simulink model "modelo_robot_6dof_dininv"  (R2023b)
settings: Solver=ode45  StartTime=0.0  StopTime=tsim  FixedStep=tstep  MaxStep=tstep
undefined symbols (not defined in the file): robot_params, tr_ref
(part 1 of 2)
settings Model: Creator=HP  LastModifiedBy=HP

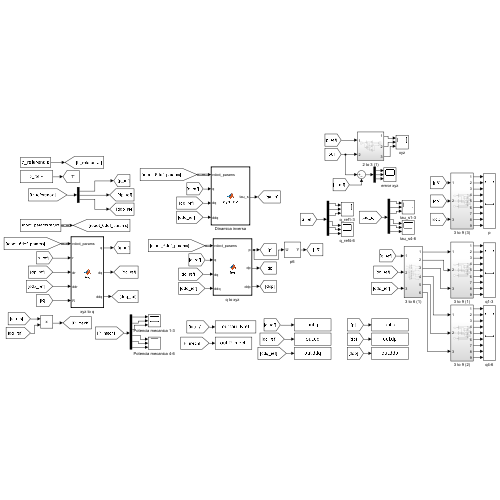
[thumbnail: Simulink's stored preview of the top-level diagram]
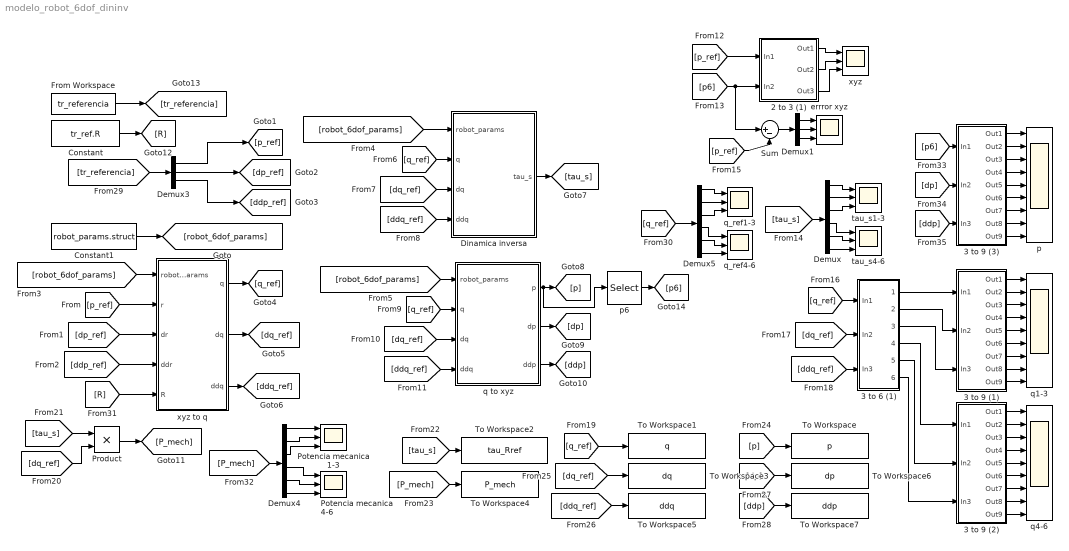
== system modelo_robot_6dof_dininv ==
  2 to 3 (1) : Subsystem
  3 to 6 (1) : Subsystem
  3 to 9 (1) : Subsystem
  3 to 9 (2) : Subsystem
  3 to 9 (3) : Subsystem
  Constant : Constant  Value=tr_ref.R
  Constant1 : Constant  Value=robot_params.struct  OutDataTypeStr=Bus: robot_params_bus
  Demux : Demux  Outputs=6
  Demux1 : Demux  Outputs=3
  Demux3 : Demux  Outputs=3
  Demux4 : Demux  Outputs=6
  Demux5 : Demux  Outputs=6
  Dinamica inversa : MATLAB Function  TreatAsAtomicUnit=on
  From Workspace : FromWorkspace  VariableName=tr_referencia
  Potencia mecanica 1-3 : Scope  NumInputPorts=3
  Potencia mecanica 4-6 : Scope  NumInputPorts=3
  Product : Product
  Sum : Sum  Inputs=|+-
  To Workspace : ToWorkspace  VariableName=p  SaveFormat=Timeseries  SampleTime=-1
  To Workspace1 : ToWorkspace  VariableName=q  SaveFormat=Timeseries  SampleTime=-1
  To Workspace2 : ToWorkspace  VariableName=tau_Rref  SaveFormat=Timeseries  SampleTime=-1
  To Workspace3 : ToWorkspace  VariableName=dq  SaveFormat=Timeseries  SampleTime=-1
  To Workspace4 : ToWorkspace  VariableName=P_mech  SaveFormat=Timeseries  SampleTime=-1
  To Workspace5 : ToWorkspace  VariableName=ddq  SaveFormat=Timeseries  SampleTime=-1
  To Workspace6 : ToWorkspace  VariableName=dp  SaveFormat=Timeseries  SampleTime=-1
  To Workspace7 : ToWorkspace  VariableName=ddp  SaveFormat=Timeseries  SampleTime=-1
  errror xyz : Scope  NumInputPorts=3
  p : Scope  NumInputPorts=9
  p6 : Selector  NumberOfDimensions=2  InputPortWidth=3  IndexOptions=Index vector (dialog),Index vector (dialog)  Indices=[1:3],3  OutputSizes=1,1
  q to xyz : MATLAB Function  TreatAsAtomicUnit=on
  q1-3 : Scope  NumInputPorts=9
  q4-6 : Scope  NumInputPorts=9
  q_ref1-3 : Scope  NumInputPorts=3
  q_ref4-6 : Scope  NumInputPorts=3
  tau_s1-3 : Scope  NumInputPorts=3
  tau_s4-6 : Scope  NumInputPorts=3
  xyz : Scope  NumInputPorts=3
  xyz to q : MATLAB Function  TreatAsAtomicUnit=on
  wires:
  Constant1/1 -> [robot_6dof_params]
  [robot_6dof_params] -> xyz to q/1(robot_params)
  [robot_6dof_params] -> Dinamica inversa/1(robot_params)
  [robot_6dof_params] -> q to xyz/1(robot_params)
  [p_ref] -> xyz to q/2(r)
  [dp_ref] -> xyz to q/3(dr)
  [ddp_ref] -> xyz to q/4(ddr)
  xyz to q/1(q) -> [q_ref]
  xyz to q/2(dq) -> [dq_ref]
  xyz to q/3(ddq) -> [ddq_ref]
  [q_ref] -> Dinamica inversa/2(q)
  [dq_ref] -> Dinamica inversa/3(dq)
  [ddq_ref] -> Dinamica inversa/4(ddq)
  [q_ref] -> q to xyz/2(q)
  [dq_ref] -> q to xyz/3(dq)
  [ddq_ref] -> q to xyz/4(ddq)
  Dinamica inversa/1(tau_s) -> [tau_s]
  q to xyz/3(ddp) -> [ddp]
  q to xyz/2(dp) -> [dp]
  [p_ref] -> 2 to 3 (1)/1(In1)
  2 to 3 (1)/1(Out1) -> xyz/1
  2 to 3 (1)/2(Out2) -> xyz/2
  2 to 3 (1)/3(Out3) -> xyz/3
  [tau_s] -> Demux/1
  Demux/1 -> tau_s1-3/1
  Demux/2 -> tau_s1-3/2
  Demux/3 -> tau_s1-3/3
  [p_ref] -> Sum/2
  Sum/1 -> Demux1/1
  Demux1/1 -> errror xyz/1
  Demux1/2 -> errror xyz/2
  Demux1/3 -> errror xyz/3
  [p6] -> Sum/1, 2 to 3 (1)/2(In2)
  3 to 9 (1)/1(Out1) -> q1-3/1
  3 to 9 (1)/2(Out2) -> q1-3/2
  3 to 9 (1)/3(Out3) -> q1-3/3
  3 to 9 (1)/4(Out4) -> q1-3/4
  3 to 9 (1)/5(Out5) -> q1-3/5
  3 to 9 (1)/6(Out6) -> q1-3/6
  3 to 9 (1)/7(Out7) -> q1-3/7
  3 to 9 (1)/8(Out8) -> q1-3/8
  3 to 9 (1)/9(Out9) -> q1-3/9
  [tau_s] -> Product/1
  [dq_ref] -> Product/2
  [q_ref] -> To Workspace1/1
  [tau_s] -> To Workspace2/1
  Product/1 -> [P_mech]
  [P_mech] -> To Workspace4/1
  [p] -> To Workspace/1
  [dq_ref] -> To Workspace3/1
  [ddq_ref] -> To Workspace5/1
  [dp] -> To Workspace6/1
  [ddp] -> To Workspace7/1
  [tr_referencia] -> Demux3/1
  From Workspace/1 -> [tr_referencia]
  Demux3/1 -> [p_ref]
  Demux3/2 -> [dp_ref]
  Demux3/3 -> [ddp_ref]
  Constant/1 -> [R]
  [R] -> xyz to q/5(R)
  Demux/4 -> tau_s4-6/1
  Demux/5 -> tau_s4-6/2
  Demux/6 -> tau_s4-6/3
  Demux5/1 -> q_ref1-3/1
  Demux5/3 -> q_ref1-3/3
  Demux5/4 -> q_ref4-6/1
  Demux5/5 -> q_ref4-6/2
  Demux5/2 -> q_ref1-3/2
  Demux5/6 -> q_ref4-6/3
  [q_ref] -> Demux5/1
  3 to 9 (2)/1(Out1) -> q4-6/1
  3 to 9 (2)/9(Out9) -> q4-6/9
  3 to 9 (2)/4(Out4) -> q4-6/4
  3 to 9 (2)/6(Out6) -> q4-6/6
  3 to 9 (2)/8(Out8) -> q4-6/8
  3 to 9 (2)/7(Out7) -> q4-6/7
  3 to 9 (2)/3(Out3) -> q4-6/3
  3 to 9 (2)/2(Out2) -> q4-6/2
  3 to 9 (2)/5(Out5) -> q4-6/5
  [q_ref] -> 3 to 6 (1)/1(In1)
  [dq_ref] -> 3 to 6 (1)/2(In2)
  [ddq_ref] -> 3 to 6 (1)/3(In3)
  3 to 6 (1)/1(Out1) -> 3 to 9 (1)/1(In1)
  3 to 6 (1)/2(Out2) -> 3 to 9 (1)/2(In2)
  3 to 6 (1)/3(Out3) -> 3 to 9 (1)/3(In3)
  3 to 6 (1)/4(Out4) -> 3 to 9 (2)/1(In1)
  3 to 6 (1)/5(Out5) -> 3 to 9 (2)/2(In2)
  3 to 6 (1)/6(Out6) -> 3 to 9 (2)/3(In3)
  Demux4/1 -> Potencia mecanica 1-3/1
  Demux4/2 -> Potencia mecanica 1-3/2
  Demux4/3 -> Potencia mecanica 1-3/3
  Demux4/4 -> Potencia mecanica 4-6/1
  Demux4/5 -> Potencia mecanica 4-6/2
  Demux4/6 -> Potencia mecanica 4-6/3
  [P_mech] -> Demux4/1
  p6/1 -> [p6]
  q to xyz/1(p) -> p6/1, [p]
  [p6] -> 3 to 9 (3)/1(In1)
  3 to 9 (3)/7(Out7) -> p/7
  3 to 9 (3)/8(Out8) -> p/8
  3 to 9 (3)/5(Out5) -> p/5
  3 to 9 (3)/1(Out1) -> p/1
  3 to 9 (3)/3(Out3) -> p/3
  3 to 9 (3)/4(Out4) -> p/4
  3 to 9 (3)/9(Out9) -> p/9
  3 to 9 (3)/2(Out2) -> p/2
  [dp] -> 3 to 9 (3)/2(In2)
  [ddp] -> 3 to 9 (3)/3(In3)
  3 to 9 (3)/6(Out6) -> p/6

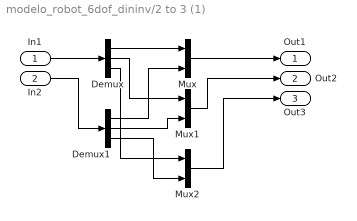
== system modelo_robot_6dof_dininv/2 to 3 (1) ==
  In1 : Inport
  In2 : Inport  Port=2
  Demux : Demux  Outputs=3
  Demux1 : Demux  Outputs=3
  Mux : Mux  Inputs=2
  Mux1 : Mux  Inputs=2
  Mux2 : Mux  Inputs=2
  Out1 : Outport
  Out2 : Outport  Port=2
  Out3 : Outport  Port=3
  wires:
  Demux/3 -> Mux2/1
  Mux2/1 -> Out3/1
  Mux1/1 -> Out2/1
  Demux/1 -> Mux/1
  Demux1/1 -> Mux/2
  In1/1 -> Demux/1
  Demux/2 -> Mux1/1
  Demux1/2 -> Mux1/2
  Mux/1 -> Out1/1
  Demux1/3 -> Mux2/2
  In2/1 -> Demux1/1

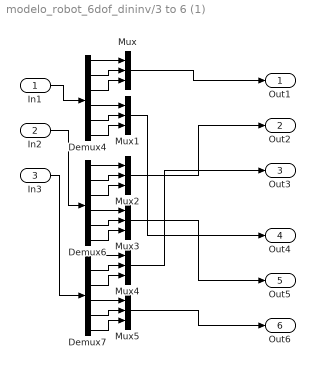
== system modelo_robot_6dof_dininv/3 to 6 (1) ==
  In1 : Inport
  In2 : Inport  Port=2
  In3 : Inport  Port=3
  Demux4 : Demux  Outputs=6
  Demux6 : Demux  Outputs=6
  Demux7 : Demux  Outputs=6
  Mux{,1..5} (6 alike) : Mux  Inputs=3
  Out1 : Outport
  Out2 : Outport  Port=2
  Out3 : Outport  Port=3
  Out4 : Outport  Port=4
  Out5 : Outport  Port=5
  Out6 : Outport  Port=6
  wires:
  Demux6/1 -> Mux2/1
  Demux6/3 -> Mux2/3
  Demux4/2 -> Mux/2
  Demux6/6 -> Mux3/3
  Demux6/2 -> Mux2/2
  Demux6/5 -> Mux3/2
  Mux/1 -> Out1/1
  In1/1 -> Demux4/1
  Demux6/4 -> Mux3/1
  Demux4/1 -> Mux/1
  Demux4/6 -> Mux1/3
  Demux4/4 -> Mux1/1
  Demux7/5 -> Mux5/2
  Demux4/3 -> Mux/3
  Demux4/5 -> Mux1/2
  Demux7/3 -> Mux4/3
  Demux7/1 -> Mux4/1
  Demux7/2 -> Mux4/2
  In3/1 -> Demux7/1
  Mux2/1 -> Out2/1
  Demux7/4 -> Mux5/1
  Demux7/6 -> Mux5/3
  In2/1 -> Demux6/1
  Mux5/1 -> Out6/1
  Mux1/1 -> Out4/1
  Mux4/1 -> Out3/1
  Mux3/1 -> Out5/1

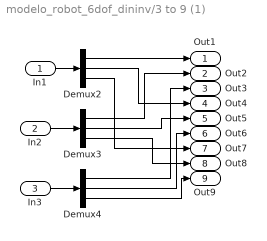
== system modelo_robot_6dof_dininv/3 to 9 (1) ==
  In1 : Inport
  In2 : Inport  Port=2
  In3 : Inport  Port=3
  Demux2 : Demux  Outputs=3
  Demux3 : Demux  Outputs=3
  Demux4 : Demux  Outputs=3
  Out1 : Outport
  Out2 : Outport  Port=2
  Out3 : Outport  Port=3
  Out4 : Outport  Port=4
  Out5 : Outport  Port=5
  Out6 : Outport  Port=6
  Out7 : Outport  Port=7
  Out8 : Outport  Port=8
  Out9 : Outport  Port=9
  wires:
  In3/1 -> Demux4/1
  Demux4/1 -> Out3/1
  Demux2/1 -> Out1/1
  Demux3/3 -> Out8/1
  Demux3/2 -> Out5/1
  Demux3/1 -> Out2/1
  In1/1 -> Demux2/1
  Demux2/3 -> Out7/1
  Demux4/3 -> Out9/1
  Demux4/2 -> Out6/1
  Demux2/2 -> Out4/1
  In2/1 -> Demux3/1

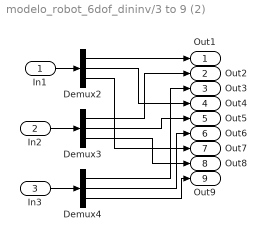
== system modelo_robot_6dof_dininv/3 to 9 (2) ==
  In1 : Inport
  In2 : Inport  Port=2
  In3 : Inport  Port=3
  Demux2 : Demux  Outputs=3
  Demux3 : Demux  Outputs=3
  Demux4 : Demux  Outputs=3
  Out1 : Outport
  Out2 : Outport  Port=2
  Out3 : Outport  Port=3
  Out4 : Outport  Port=4
  Out5 : Outport  Port=5
  Out6 : Outport  Port=6
  Out7 : Outport  Port=7
  Out8 : Outport  Port=8
  Out9 : Outport  Port=9
  wires:
  In3/1 -> Demux4/1
  Demux4/1 -> Out3/1
  Demux2/1 -> Out1/1
  Demux3/3 -> Out8/1
  Demux3/2 -> Out5/1
  Demux3/1 -> Out2/1
  In1/1 -> Demux2/1
  Demux2/3 -> Out7/1
  Demux4/3 -> Out9/1
  Demux4/2 -> Out6/1
  Demux2/2 -> Out4/1
  In2/1 -> Demux3/1

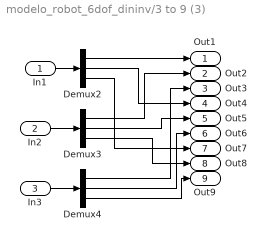
== system modelo_robot_6dof_dininv/3 to 9 (3) ==
  In1 : Inport
  In2 : Inport  Port=2
  In3 : Inport  Port=3
  Demux2 : Demux  Outputs=3
  Demux3 : Demux  Outputs=3
  Demux4 : Demux  Outputs=3
  Out1 : Outport
  Out2 : Outport  Port=2
  Out3 : Outport  Port=3
  Out4 : Outport  Port=4
  Out5 : Outport  Port=5
  Out6 : Outport  Port=6
  Out7 : Outport  Port=7
  Out8 : Outport  Port=8
  Out9 : Outport  Port=9
  wires:
  In3/1 -> Demux4/1
  Demux4/1 -> Out3/1
  Demux2/1 -> Out1/1
  Demux3/3 -> Out8/1
  Demux3/2 -> Out5/1
  Demux3/1 -> Out2/1
  In1/1 -> Demux2/1
  Demux2/3 -> Out7/1
  Demux4/3 -> Out9/1
  Demux4/2 -> Out6/1
  Demux2/2 -> Out4/1
  In2/1 -> Demux3/1

== matlab function modelo_robot_6dof_dininv/xyz to q ==
  data: robot_params input; q output size=[6,1]; r input size=[3,1]; dr input size=[3,1]; ddr input size=[3,1]; dq output size=[6,1]; ddq output size=[6,1]; R input size=[3,3]
function [q,dq,ddq] = fcn(robot_params,r,dr,ddr,R)

%l1 = robot_params.l(1);
l2 = robot_params.l(2);
l3 = robot_params.l(3);
%l4 = robot_params.l(4);
%l5 = robot_params.l(5);
%l6 = robot_params.l(6);

lc1 = robot_params.lc(1);
lc2 = robot_params.lc(2);
lc3 = robot_params.lc(3);
%lc4 = robot_params.lc(4);
%lc5 = robot_params.lc(5);
%lc6 = robot_params.lc(6);

d1 = robot_params.d(1);
%d2 = robot_params.d(2);
%d3 = robot_params.d(3);
d4 = robot_params.d(4);
d5 = robot_params.d(5);
d6 = robot_params.d(6);

dc1 = robot_params.dc(1);
%dc2 = robot_params.dc(2);
%dc3 = robot_params.dc(3);
dc4 = robot_params.dc(4);
dc5 = robot_params.dc(5);
dc6 = robot_params.dc(6);

Xr = r(1);
Yr = r(2);
Zr = r(3);

% Cinematica inversa %%%%%%%%%%%%%%%%%%%%%%%%%%%%%%%%%%%%%%%%%%%%%%%%%%%%%%

A = d6*R(2,3) - Yr;
B = Xr - d6*R(1,3);

q1 = + atan2(sqrt(B^2+A^2-d4^2),d4) + atan2(B,A); %signo

c1 = cos(q1);
s1 = sin(q1);

C = c1*R(1,1) + s1*R(2,1);
D = c1*R(2,2) - s1*R(1,2);
E = s1*R(1,1) - c1*R(2,1);

q5 = + atan2(sqrt(E^2+D^2),s1*R(1,3)-c1*R(2,3)); %signo

c5 = cos(q5);
s5 = sin(q5);

q6 = atan2(D/s5,E/s5);

c6 = cos(q6);
s6 = sin(q6);

F = c5*c6;  

q234 = atan2(R(3,1)*F-s6*C,F*C+s6*R(3,1));

c234 = cos(q234);
s234 = sin(q234);

KC = c1*Xr + s1*Yr - s234*d5 + c234*s5*d6;
KS = Zr - d1 + c234*d5 + s234*s5*d6;

c3 = (KS^2 + KC^2 - l2^2 - l3^2)/(2*l2*l3);
s3 = sqrt(1-c3^2);

q3 = + atan2(s3,c3); %signo %no cambiar
q2 = atan2(KS,KC) - atan2(s3*l3,c3*l3+l2);
q4 = q234 - q2 - q3;


q = [q1;q2;q3;q4;q5;q6];

% Cinematica diferencial %%%%%%%%%%%%%%%%%%%%%%%%%%%%%%%%%%%%%%%%%%%%%%%%%%

JP = zeros(3,6);

JP(1,1) = -cos(q1)*(d1 + l3*sin(q2 + q3) + l2*sin(q2) - d5*cos(q2 + q3 + q4) - dc6*sin(q2 + q3 + q4)*sin(q5));
JP(1,2) = -cos(q1)*(d1 - dc1 + l3*sin(q2 + q3) + l2*sin(q2) - d5*cos(q2 + q3 + q4) - dc6*sin(q2 + q3 + q4)*sin(q5));
JP(1,3) = cos(q1)*(lc2*sin(q2) - l2*sin(q2) - l3*sin(q2 + q3) + d5*cos(q2 + q3 + q4) + dc6*sin(q2 + q3 + q4)*sin(q5));
JP(1,4) = - cos(q2 + q3 + q4)*(dc6*(cos(q1)*cos(q5) + cos(q2 + q3 + q4)*sin(q1)*sin(q5)) + d4*cos(q1) - sin(q1)*(l3*cos(q2 + q3) + l2*cos(q2)) + sin(q1)*(lc3*cos(q2 + q3) + l2*cos(q2)) - d5*sin(q2 + q3 + q4)*sin(q1)) - sin(q2 + q3 + q4)*sin(q1)*(lc3*sin(q2 + q3) - l3*sin(q2 + q3) + d5*cos(q2 + q3 + q4) + dc6*sin(q2 + q3 + q4)*sin(q5));
JP(1,5) = d5*sin(q1)*sin(q5) + d5*cos(q2 + q3 + q4)*cos(q1)*cos(q5) - d4*sin(q2 + q3 + q4)*cos(q1)*sin(q5) + dc4*sin(q2 + q3 + q4)*cos(q1)*sin(q5);
JP(1,6) = (d5 - dc5)*(sin(q1)*sin(q5) + cos(q2 + q3 + q4)*cos(q1)*cos(q5));

JP(2,1) = -sin(q1)*(d1 + l3*sin(q2 + q3) + l2*sin(q2) - d5*cos(q2 + q3 + q4) - dc6*sin(q2 + q3 + q4)*sin(q5));
JP(2,2) = -sin(q1)*(d1 - dc1 + l3*sin(q2 + q3) + l2*sin(q2) - d5*cos(q2 + q3 + q4) - dc6*sin(q2 + q3 + q4)*sin(q5));
JP(2,3) = sin(q1)*(lc2*sin(q2) - l2*sin(q2) - l3*sin(q2 + q3) + d5*cos(q2 + q3 + q4) + dc6*sin(q2 + q3 + q4)*sin(q5));
JP(2,4) = sin(q2 + q3 + q4)*cos(q1)*(lc3*sin(q2 + q3) - l3*sin(q2 + q3) + d5*cos(q2 + q3 + q4) + dc6*sin(q2 + q3 + q4)*sin(q5)) - cos(q2 + q3 + q4)*(dc6*(cos(q5)*sin(q1) - cos(q2 + q3 + q4)*cos(q1)*sin(q5)) + cos(q1)*(l3*cos(q2 + q3) + l2*cos(q2)) - cos(q1)*(lc3*cos(q2 + q3) + l2*cos(q2)) + d4*sin(q1) + d5*sin(q2 + q3 + q4)*cos(q1));
JP(2,5) = d5*cos(q2 + q3 + q4)*cos(q5)*sin(q1) - d5*cos(q1)*sin(q5) - d4*sin(q2 + q3 + q4)*sin(q1)*sin(q5) + dc4*sin(q2 + q3 + q4)*sin(q1)*sin(q5);
JP(2,6) = -(d5 - dc5)*(cos(q1)*sin(q5) - cos(q2 + q3 + q4)*cos(q5)*sin(q1));

JP(3,1) = l3*cos(q2 + q3) - (dc6*sin(q2 + q3 + q4 + q5))/2 + l2*cos(q2) + (dc6*sin(q2 + q3 + q4 - q5))/2 + d5*sin(q2 + q3 + q4);
JP(3,2) = l3*cos(q2 + q3) - (dc6*sin(q2 + q3 + q4 + q5))/2 - lc1 + l2*cos(q2) + (dc6*sin(q2 + q3 + q4 - q5))/2 + d5*sin(q2 + q3 + q4);
JP(3,3) = l3*cos(q2 + q3) - (dc6*sin(q2 + q3 + q4 + q5))/2 + l2*cos(q2) - lc2*cos(q2) + (dc6*sin(q2 + q3 + q4 - q5))/2 + d5*sin(q2 + q3 + q4);
JP(3,4) = - (dc6*sin(q2 + q3 + q4 + q5))/2 - (dc6*sin(q2 + q3 + q4 - q5))/2 - d4*sin(q2 + q3 + q4);
JP(3,5) = d4*cos(q2 + q3 + q4)*sin(q5) + d5*sin(q2 + q3 + q4)*cos(q5) - dc4*cos(q2 + q3 + q4)*sin(q5);
JP(3,6) = sin(q2 + q3 + q4)*cos(q5)*(d5 - dc5);

% Pseudoinversa derecha JPinv = zeros(6,3)
JPinv = JP.'*(JP*JP.')^-1;

% Velocidades articulares
dq = JPinv*dr;

dq1 = dq(1);
dq2 = dq(2);
dq3 = dq(3);
dq4 = dq(4);
dq5 = dq(5);
%dq6 = dq(6);

dJP = zeros(3,6);

dJP(1,1) = dq1*sin(q1)*(d1 + l3*sin(q2 + q3) + l2*sin(q2) - d5*cos(q2 + q3 + q4) - dc6*sin(q2 + q3 + q4)*sin(q5)) - dq3*cos(q1)*(l3*cos(q2 + q3) + d5*sin(q2 + q3 + q4) - dc6*cos(q2 + q3 + q4)*sin(q5)) - dq4*cos(q1)*(d5*sin(q2 + q3 + q4) - dc6*cos(q2 + q3 + q4)*sin(q5)) - dq2*cos(q1)*(l3*cos(q2 + q3) + l2*cos(q2) + d5*sin(q2 + q3 + q4) - dc6*cos(q2 + q3 + q4)*sin(q5)) + dc6*dq5*sin(q2 + q3 + q4)*cos(q1)*cos(q5);
dJP(1,2) = dq1*sin(q1)*(d1 - dc1 + l3*sin(q2 + q3) + l2*sin(q2) - d5*cos(q2 + q3 + q4) - dc6*sin(q2 + q3 + q4)*sin(q5)) - dq3*cos(q1)*(l3*cos(q2 + q3) + d5*sin(q2 + q3 + q4) - dc6*cos(q2 + q3 + q4)*sin(q5)) - dq4*cos(q1)*(d5*sin(q2 + q3 + q4) - dc6*cos(q2 + q3 + q4)*sin(q5)) - dq2*cos(q1)*(l3*cos(q2 + q3) + l2*cos(q2) + d5*sin(q2 + q3 + q4) - dc6*cos(q2 + q3 + q4)*sin(q5)) + dc6*dq5*sin(q2 + q3 + q4)*cos(q1)*cos(q5);
dJP(1,3) = dc6*dq5*sin(q2 + q3 + q4)*cos(q1)*cos(q5) - dq2*cos(q1)*(l3*cos(q2 + q3) + l2*cos(q2) - lc2*cos(q2) + d5*sin(q2 + q3 + q4) - dc6*cos(q2 + q3 + q4)*sin(q5)) - dq1*sin(q1)*(lc2*sin(q2) - l2*sin(q2) - l3*sin(q2 + q3) + d5*cos(q2 + q3 + q4) + dc6*sin(q2 + q3 + q4)*sin(q5)) - dq4*cos(q1)*(d5*sin(q2 + q3 + q4) - dc6*cos(q2 + q3 + q4)*sin(q5)) - dq3*cos(q1)*(l3*cos(q2 + q3) + d5*sin(q2 + q3 + q4) - dc6*cos(q2 + q3 + q4)*sin(q5));
dJP(1,4) = dq1*l3*cos(q1)*cos(q4) - dq1*lc3*cos(q1)*cos(q4) - dc6*dq1*cos(q1)*sin(q5) - dc6*dq5*cos(q5)*sin(q1) - dq4*l3*sin(q1)*sin(q4) + dq4*lc3*sin(q1)*sin(q4) + d4*dq1*cos(q2)*cos(q3)*cos(q4)*sin(q1) + d4*dq2*cos(q1)*cos(q2)*cos(q3)*sin(q4) + d4*dq2*cos(q1)*cos(q2)*cos(q4)*sin(q3) + d4*dq2*cos(q1)*cos(q3)*cos(q4)*sin(q2) + d4*dq3*cos(q1)*cos(q2)*cos(q3)*sin(q4) + d4*dq3*cos(q1)*cos(q2)*cos(q4)*sin(q3) + d4*dq3*cos(q1)*cos(q3)*cos(q4)*sin(q2) + d4*dq4*cos(q1)*cos(q2)*cos(q3)*sin(q4) + d4*dq4*cos(q1)*cos(q2)*cos(q4)*sin(q3) + d4*dq4*cos(q1)*cos(q3)*cos(q4)*sin(q2) - d4*dq1*cos(q2)*sin(q1)*sin(q3)*sin(q4) - d4*dq1*cos(q3)*sin(q1)*sin(q2)*sin(q4) - d4*dq1*cos(q4)*sin(q1)*sin(q2)*sin(q3) - d4*dq2*cos(q1)*sin(q2)*sin(q3)*sin(q4) - d4*dq3*cos(q1)*sin(q2)*sin(q3)*sin(q4) - d4*dq4*cos(q1)*sin(q2)*sin(q3)*sin(q4) + dc6*dq1*cos(q2)*cos(q3)*cos(q4)*cos(q5)*sin(q1) + dc6*dq2*cos(q1)*cos(q2)*cos(q3)*cos(q5)*sin(q4) + dc6*dq2*cos(q1)*cos(q2)*cos(q4)*cos(q5)*sin(q3) + dc6*dq2*cos(q1)*cos(q3)*cos(q4)*cos(q5)*sin(q2) + dc6*dq3*cos(q1)*cos(q2)*cos(q3)*cos(q5)*sin(q4) + dc6*dq3*cos(q1)*cos(q2)*cos(q4)*cos(q5)*sin(q3) + dc6*dq3*cos(q1)*cos(q3)*cos(q4)*cos(q5)*sin(q2) + dc6*dq4*cos(q1)*cos(q2)*cos(q3)*cos(q5)*sin(q4) + dc6*dq4*cos(q1)*cos(q2)*cos(q4)*cos(q5)*sin(q3) + dc6*dq4*cos(q1)*cos(q3)*cos(q4)*cos(q5)*sin(q2) + dc6*dq5*cos(q1)*cos(q2)*cos(q3)*cos(q4)*sin(q5) - dc6*dq1*cos(q2)*cos(q5)*sin(q1)*sin(q3)*sin(q4) - dc6*dq1*cos(q3)*cos(q5)*sin(q1)*sin(q2)*sin(q4) - dc6*dq1*cos(q4)*cos(q5)*sin(q1)*sin(q2)*sin(q3) - dc6*dq2*cos(q1)*cos(q5)*sin(q2)*sin(q3)*sin(q4) - dc6*dq3*cos(q1)*cos(q5)*sin(q2)*sin(q3)*sin(q4) - dc6*dq4*cos(q1)*cos(q5)*sin(q2)*sin(q3)*sin(q4) - dc6*dq5*cos(q1)*cos(q2)*sin(q3)*sin(q4)*sin(q5) - dc6*dq5*cos(q1)*cos(q3)*sin(q2)*sin(q4)*sin(q5) - dc6*dq5*cos(q1)*cos(q4)*sin(q2)*sin(q3)*sin(q5);
dJP(1,5) = dq5*(d5*cos(q5)*sin(q1) - d4*sin(q2 + q3 + q4)*cos(q1)*cos(q5) - d5*cos(q2 + q3 + q4)*cos(q1)*sin(q5) + dc4*sin(q2 + q3 + q4)*cos(q1)*cos(q5)) + dq1*(d5*cos(q1)*sin(q5) - d5*cos(q2 + q3 + q4)*cos(q5)*sin(q1) + d4*sin(q2 + q3 + q4)*sin(q1)*sin(q5) - dc4*sin(q2 + q3 + q4)*sin(q1)*sin(q5)) - dq2*cos(q1)*(d4*cos(q2 + q3 + q4)*sin(q5) + d5*sin(q2 + q3 + q4)*cos(q5) - dc4*cos(q2 + q3 + q4)*sin(q5)) - dq3*cos(q1)*(d4*cos(q2 + q3 + q4)*sin(q5) + d5*sin(q2 + q3 + q4)*cos(q5) - dc4*cos(q2 + q3 + q4)*sin(q5)) - dq4*cos(q1)*(d4*cos(q2 + q3 + q4)*sin(q5) + d5*sin(q2 + q3 + q4)*cos(q5) - dc4*cos(q2 + q3 + q4)*sin(q5));
dJP(1,6) = dq1*(d5 - dc5)*(cos(q1)*sin(q5) - cos(q2 + q3 + q4)*cos(q5)*sin(q1)) + dq5*(d5 - dc5)*(cos(q5)*sin(q1) - cos(q2 + q3 + q4)*cos(q1)*sin(q5)) - dq2*sin(q2 + q3 + q4)*cos(q1)*cos(q5)*(d5 - dc5) - dq3*sin(q2 + q3 + q4)*cos(q1)*cos(q5)*(d5 - dc5) - dq4*sin(q2 + q3 + q4)*cos(q1)*cos(q5)*(d5 - dc5);

dJP(2,1) = dc6*dq5*sin(q2 + q3 + q4)*cos(q5)*sin(q1) - dq1*cos(q1)*(d1 + l3*sin(q2 + q3) + l2*sin(q2) - d5*cos(q2 + q3 + q4) - dc6*sin(q2 + q3 + q4)*sin(q5)) - dq4*sin(q1)*(d5*sin(q2 + q3 + q4) - dc6*cos(q2 + q3 + q4)*sin(q5)) - dq2*sin(q1)*(l3*cos(q2 + q3) + l2*cos(q2) + d5*sin(q2 + q3 + q4) - dc6*cos(q2 + q3 + q4)*sin(q5)) - dq3*sin(q1)*(l3*cos(q2 + q3) + d5*sin(q2 + q3 + q4) - dc6*cos(q2 + q3 + q4)*sin(q5));
dJP(2,2) = dc6*dq5*sin(q2 + q3 + q4)*cos(q5)*sin(q1) - dq4*sin(q1)*(d5*sin(q2 + q3 + q4) - dc6*cos(q2 + q3 + q4)*sin(q5)) - dq2*sin(q1)*(l3*cos(q2 + q3) + l2*cos(q2) + d5*sin(q2 + q3 + q4) - dc6*cos(q2 + q3 + q4)*sin(q5)) - dq1*cos(q1)*(d1 - dc1 + l3*sin(q2 + q3) + l2*sin(q2) - d5*cos(q2 + q3 + q4) - dc6*sin(q2 + q3 + q4)*sin(q5)) - dq3*sin(q1)*(l3*cos(q2 + q3) + d5*sin(q2 + q3 + q4) - dc6*cos(q2 + q3 + q4)*sin(q5));
dJP(2,3) = dq1*cos(q1)*(lc2*sin(q2) - l2*sin(q2) - l3*sin(q2 + q3) + d5*cos(q2 + q3 + q4) + dc6*sin(q2 + q3 + q4)*sin(q5)) - dq2*sin(q1)*(l3*cos(q2 + q3) + l2*cos(q2) - lc2*cos(q2) + d5*sin(q2 + q3 + q4) - dc6*cos(q2 + q3 + q4)*sin(q5)) - dq3*sin(q1)*(l3*cos(q2 + q3) + d5*sin(q2 + q3 + q4) - dc6*cos(q2 + q3 + q4)*sin(q5)) - dq4*sin(q1)*(d5*sin(q2 + q3 + q4) - dc6*cos(q2 + q3 + q4)*sin(q5)) + dc6*dq5*sin(q2 + q3 + q4)*cos(q5)*sin(q1);
dJP(2,4) = dc6*dq5*cos(q1)*cos(q5) + dq1*l3*cos(q4)*sin(q1) + dq4*l3*cos(q1)*sin(q4) - dq1*lc3*cos(q4)*sin(q1) - dq4*lc3*cos(q1)*sin(q4) - dc6*dq1*sin(q1)*sin(q5) - d4*dq1*cos(q1)*cos(q2)*cos(q3)*cos(q4) + d4*dq1*cos(q1)*cos(q2)*sin(q3)*sin(q4) + d4*dq1*cos(q1)*cos(q3)*sin(q2)*sin(q4) + d4*dq1*cos(q1)*cos(q4)*sin(q2)*sin(q3) + d4*dq2*cos(q2)*cos(q3)*sin(q1)*sin(q4) + d4*dq2*cos(q2)*cos(q4)*sin(q1)*sin(q3) + d4*dq2*cos(q3)*cos(q4)*sin(q1)*sin(q2) + d4*dq3*cos(q2)*cos(q3)*sin(q1)*sin(q4) + d4*dq3*cos(q2)*cos(q4)*sin(q1)*sin(q3) + d4*dq3*cos(q3)*cos(q4)*sin(q1)*sin(q2) + d4*dq4*cos(q2)*cos(q3)*sin(q1)*sin(q4) + d4*dq4*cos(q2)*cos(q4)*sin(q1)*sin(q3) + d4*dq4*cos(q3)*cos(q4)*sin(q1)*sin(q2) - d4*dq2*sin(q1)*sin(q2)*sin(q3)*sin(q4) - d4*dq3*sin(q1)*sin(q2)*sin(q3)*sin(q4) - d4*dq4*sin(q1)*sin(q2)*sin(q3)*sin(q4) - dc6*dq1*cos(q1)*cos(q2)*cos(q3)*cos(q4)*cos(q5) + dc6*dq1*cos(q1)*cos(q2)*cos(q5)*sin(q3)*sin(q4) + dc6*dq1*cos(q1)*cos(q3)*cos(q5)*sin(q2)*sin(q4) + dc6*dq1*cos(q1)*cos(q4)*cos(q5)*sin(q2)*sin(q3) + dc6*dq2*cos(q2)*cos(q3)*cos(q5)*sin(q1)*sin(q4) + dc6*dq2*cos(q2)*cos(q4)*cos(q5)*sin(q1)*sin(q3) + dc6*dq2*cos(q3)*cos(q4)*cos(q5)*sin(q1)*sin(q2) + dc6*dq3*cos(q2)*cos(q3)*cos(q5)*sin(q1)*sin(q4) + dc6*dq3*cos(q2)*cos(q4)*cos(q5)*sin(q1)*sin(q3) + dc6*dq3*cos(q3)*cos(q4)*cos(q5)*sin(q1)*sin(q2) + dc6*dq4*cos(q2)*cos(q3)*cos(q5)*sin(q1)*sin(q4) + dc6*dq4*cos(q2)*cos(q4)*cos(q5)*sin(q1)*sin(q3) + dc6*dq4*cos(q3)*cos(q4)*cos(q5)*sin(q1)*sin(q2) + dc6*dq5*cos(q2)*cos(q3)*cos(q4)*sin(q1)*sin(q5) - dc6*dq2*cos(q5)*sin(q1)*sin(q2)*sin(q3)*sin(q4) - dc6*dq3*cos(q5)*sin(q1)*sin(q2)*sin(q3)*sin(q4) - dc6*dq4*cos(q5)*sin(q1)*sin(q2)*sin(q3)*sin(q4) - dc6*dq5*cos(q2)*sin(q1)*sin(q3)*sin(q4)*sin(q5) - dc6*dq5*cos(q3)*sin(q1)*sin(q2)*sin(q4)*sin(q5) - dc6*dq5*cos(q4)*sin(q1)*sin(q2)*sin(q3)*sin(q5);
dJP(2,5) = dq1*(d5*sin(q1)*sin(q5) + d5*cos(q2 + q3 + q4)*cos(q1)*cos(q5) - d4*sin(q2 + q3 + q4)*cos(q1)*sin(q5) + dc4*sin(q2 + q3 + q4)*cos(q1)*sin(q5)) - dq5*(d5*cos(q1)*cos(q5) + d4*sin(q2 + q3 + q4)*cos(q5)*sin(q1) + d5*cos(q2 + q3 + q4)*sin(q1)*sin(q5) - dc4*sin(q2 + q3 + q4)*cos(q5)*sin(q1)) - dq2*sin(q1)*(d4*cos(q2 + q3 + q4)*sin(q5) + d5*sin(q2 + q3 + q4)*cos(q5) - dc4*cos(q2 + q3 + q4)*sin(q5)) - dq3*sin(q1)*(d4*cos(q2 + q3 + q4)*sin(q5) + d5*sin(q2 + q3 + q4)*cos(q5) - dc4*cos(q2 + q3 + q4)*sin(q5)) - dq4*sin(q1)*(d4*cos(q2 + q3 + q4)*sin(q5) + d5*sin(q2 + q3 + q4)*cos(q5) - dc4*cos(q2 + q3 + q4)*sin(q5));
dJP(2,6) = dq1*(d5 - dc5)*(sin(q1)*sin(q5) + cos(q2 + q3 + q4)*cos(q1)*cos(q5)) - dq5*(d5 - dc5)*(cos(q1)*cos(q5) + cos(q2 + q3 + q4)*sin(q1)*sin(q5)) - dq2*sin(q2 + q3 + q4)*cos(q5)*sin(q1)*(d5 - dc5) - dq3*sin(q2 + q3 + q4)*cos(q5)*sin(q1)*(d5 - dc5) - dq4*sin(q2 + q3 + q4)*cos(q5)*sin(q1)*(d5 - dc5);

dJP(3,1) = dq4*((dc6*cos(q2 + q3 + q4 - q5))/2 - (dc6*cos(q2 + q3 + q4 + q5))/2 + d5*cos(q2 + q3 + q4)) - dq3*((dc6*cos(q2 + q3 + q4 + q5))/2 + l3*sin(q2 + q3) - (dc6*cos(q2 + q3 + q4 - q5))/2 - d5*cos(q2 + q3 + q4)) - dq2*((dc6*cos(q2 + q3 + q4 + q5))/2 + l3*sin(q2 + q3) - (dc6*cos(q2 + q3 + q4 - q5))/2 + l2*sin(q2) - d5*cos(q2 + q3 + q4)) - (dc6*dq5*(cos(q2 + q3 + q4 + q5) + cos(q2 + q3 + q4 - q5)))/2;
dJP(3,2) = dq4*((dc6*cos(q2 + q3 + q4 - q5))/2 - (dc6*cos(q2 + q3 + q4 + q5))/2 + d5*cos(q2 + q3 + q4)) - dq3*((dc6*cos(q2 + q3 + q4 + q5))/2 + l3*sin(q2 + q3) - (dc6*cos(q2 + q3 + q4 - q5))/2 - d5*cos(q2 + q3 + q4)) - dq2*((dc6*cos(q2 + q3 + q4 + q5))/2 + l3*sin(q2 + q3) - (dc6*cos(q2 + q3 + q4 - q5))/2 + l2*sin(q2) - d5*cos(q2 + q3 + q4)) - (dc6*dq5*(cos(q2 + q3 + q4 + q5) + cos(q2 + q3 + q4 - q5)))/2;
dJP(3,3) = dq4*((dc6*cos(q2 + q3 + q4 - q5))/2 - (dc6*cos(q2 + q3 + q4 + q5))/2 + d5*cos(q2 + q3 + q4)) - dq3*((dc6*cos(q2 + q3 + q4 + q5))/2 + l3*sin(q2 + q3) - (dc6*cos(q2 + q3 + q4 - q5))/2 - d5*cos(q2 + q3 + q4)) - dq2*((dc6*cos(q2 + q3 + q4 + q5))/2 + l3*sin(q2 + q3) - (dc6*cos(q2 + q3 + q4 - q5))/2 + l2*sin(q2) - lc2*sin(q2) - d5*cos(q2 + q3 + q4)) - dq5*((dc6*cos(q2 + q3 + q4 + q5))/2 + (dc6*cos(q2 + q3 + q4 - q5))/2);
dJP(3,4) = - dq2*((dc6*cos(q2 + q3 + q4 + q5))/2 + (dc6*cos(q2 + q3 + q4 - q5))/2 + d4*cos(q2 + q3 + q4)) - dq3*((dc6*cos(q2 + q3 + q4 + q5))/2 + (dc6*cos(q2 + q3 + q4 - q5))/2 + d4*cos(q2 + q3 + q4)) - dq4*((dc6*cos(q2 + q3 + q4 + q5))/2 + (dc6*cos(q2 + q3 + q4 - q5))/2 + d4*cos(q2 + q3 + q4)) - (dc6*dq5*(cos(q2 + q3 + q4 + q5) - cos(q2 + q3 + q4 - q5)))/2;
dJP(3,5) = dq2*(d5*cos(q2 + q3 + q4)*cos(q5) - d4*sin(q2 + q3 + q4)*sin(q5) + dc4*sin(q2 + q3 + q4)*sin(q5)) - dq5*(dc4*cos(q2 + q3 + q4)*cos(q5) - d4*cos(q2 + q3 + q4)*cos(q5) + d5*sin(q2 + q3 + q4)*sin(q5)) + dq3*(d5*cos(q2 + q3 + q4)*cos(q5) - d4*sin(q2 + q3 + q4)*sin(q5) + dc4*sin(q2 + q3 + q4)*sin(q5)) + dq4*(d5*cos(q2 + q3 + q4)*cos(q5) - d4*sin(q2 + q3 + q4)*sin(q5) + dc4*sin(q2 + q3 + q4)*sin(q5));
dJP(3,6) = (d5 - dc5)*(dq2*cos(q2 + q3 + q4)*cos(q5) + dq3*cos(q2 + q3 + q4)*cos(q5) + dq4*cos(q2 + q3 + q4)*cos(q5) - dq5*sin(q2 + q3 + q4)*sin(q5));

% Aceleraciones articulares
ddq = JPinv*(ddr - dJP*dq);

== matlab function modelo_robot_6dof_dininv/q to xyz ==
  data: robot_params input; p output size=[3,6]; q input size=[6,1]; dq input size=[6,1]; ddq input size=[6,1]; dp output size=[3,1]; ddp output size=[3,1]
function [p,dp,ddp] = fcn(robot_params,q,dq,ddq)

l1 = robot_params.l(1);
l2 = robot_params.l(2);
l3 = robot_params.l(3);
l4 = robot_params.l(4);
l5 = robot_params.l(5);
l6 = robot_params.l(6);

lc1 = robot_params.lc(1);
lc2 = robot_params.lc(2);
lc3 = robot_params.lc(3);
lc4 = robot_params.lc(4);
lc5 = robot_params.lc(5);
lc6 = robot_params.lc(6);

d1 = robot_params.d(1);
d2 = robot_params.d(2);
d3 = robot_params.d(3);
d4 = robot_params.d(4);
d5 = robot_params.d(5);
d6 = robot_params.d(6);

dc1 = robot_params.dc(1);
dc2 = robot_params.dc(2);
dc3 = robot_params.dc(3);
dc4 = robot_params.dc(4);
dc5 = robot_params.dc(5);
dc6 = robot_params.dc(6);

q1 = q(1);
q2 = q(2);
q3 = q(3);
q4 = q(4);
q5 = q(5);
q6 = q(6);


% Cinematica directa %%%%%%%%%%%%%%%%%%%%%%%%%%%%%%%%%%%%%%%%%%%%%%%%%%%%%%

DH = [0   pi/2  d1 q1;
      l2  0     0  q2;
      l3  0     0  q3;
      0   pi/2  d4 q4;
      0   -pi/2 d5 q5;
      0   0     d6 q6];

A01 = transformacion_homogenea(DH(1,:));
A12 = transformacion_homogenea(DH(2,:));
A23 = transformacion_homogenea(DH(3,:));
A34 = transformacion_homogenea(DH(4,:));
A45 = transformacion_homogenea(DH(5,:));
A56 = transformacion_homogenea(DH(6,:));

T0 = zeros(4,4,6);

T0(:,:,1) = A01;
T0(:,:,2) = A01*A12;
T0(:,:,3) = A01*A12*A23;
T0(:,:,4) = A01*A12*A23*A34;
T0(:,:,5) = A01*A12*A23*A34*A45;
T0(:,:,6) = A01*A12*A23*A34*A45*A56;

p = reshape(T0(1:3,4,:),[3,6]);


% Cinematica diferencial %%%%%%%%%%%%%%%%%%%%%%%%%%%%%%%%%%%%%%%%%%%%%%%%%%
JP = zeros(3,6);

JP(1,1) = -cos(q1)*(d1 + l3*sin(q2 + q3) + l2*sin(q2) - d5*cos(q2 + q3 + q4) - dc6*sin(q2 + q3 + q4)*sin(q5));
JP(1,2) = -cos(q1)*(d1 - dc1 + l3*sin(q2 + q3) + l2*sin(q2) - d5*cos(q2 + q3 + q4) - dc6*sin(q2 + q3 + q4)*sin(q5));
JP(1,3) = cos(q1)*(lc2*sin(q2) - l2*sin(q2) - l3*sin(q2 + q3) + d5*cos(q2 + q3 + q4) + dc6*sin(q2 + q3 + q4)*sin(q5));
JP(1,4) = - cos(q2 + q3 + q4)*(dc6*(cos(q1)*cos(q5) + cos(q2 + q3 + q4)*sin(q1)*sin(q5)) + d4*cos(q1) - sin(q1)*(l3*cos(q2 + q3) + l2*cos(q2)) + sin(q1)*(lc3*cos(q2 + q3) + l2*cos(q2)) - d5*sin(q2 + q3 + q4)*sin(q1)) - sin(q2 + q3 + q4)*sin(q1)*(lc3*sin(q2 + q3) - l3*sin(q2 + q3) + d5*cos(q2 + q3 + q4) + dc6*sin(q2 + q3 + q4)*sin(q5));
JP(1,5) = d5*sin(q1)*sin(q5) + d5*cos(q2 + q3 + q4)*cos(q1)*cos(q5) - d4*sin(q2 + q3 + q4)*cos(q1)*sin(q5) + dc4*sin(q2 + q3 + q4)*cos(q1)*sin(q5);
JP(1,6) = (d5 - dc5)*(sin(q1)*sin(q5) + cos(q2 + q3 + q4)*cos(q1)*cos(q5));

JP(2,1) = -sin(q1)*(d1 + l3*sin(q2 + q3) + l2*sin(q2) - d5*cos(q2 + q3 + q4) - dc6*sin(q2 + q3 + q4)*sin(q5));
JP(2,2) = -sin(q1)*(d1 - dc1 + l3*sin(q2 + q3) + l2*sin(q2) - d5*cos(q2 + q3 + q4) - dc6*sin(q2 + q3 + q4)*sin(q5));
JP(2,3) = sin(q1)*(lc2*sin(q2) - l2*sin(q2) - l3*sin(q2 + q3) + d5*cos(q2 + q3 + q4) + dc6*sin(q2 + q3 + q4)*sin(q5));
JP(2,4) = sin(q2 + q3 + q4)*cos(q1)*(lc3*sin(q2 + q3) - l3*sin(q2 + q3) + d5*cos(q2 + q3 + q4) + dc6*sin(q2 + q3 + q4)*sin(q5)) - cos(q2 + q3 + q4)*(dc6*(cos(q5)*sin(q1) - cos(q2 + q3 + q4)*cos(q1)*sin(q5)) + cos(q1)*(l3*cos(q2 + q3) + l2*cos(q2)) - cos(q1)*(lc3*cos(q2 + q3) + l2*cos(q2)) + d4*sin(q1) + d5*sin(q2 + q3 + q4)*cos(q1));
JP(2,5) = d5*cos(q2 + q3 + q4)*cos(q5)*sin(q1) - d5*cos(q1)*sin(q5) - d4*sin(q2 + q3 + q4)*sin(q1)*sin(q5) + dc4*sin(q2 + q3 + q4)*sin(q1)*sin(q5);
JP(2,6) = -(d5 - dc5)*(cos(q1)*sin(q5) - cos(q2 + q3 + q4)*cos(q5)*sin(q1));

JP(3,1) = l3*cos(q2 + q3) - (dc6*sin(q2 + q3 + q4 + q5))/2 + l2*cos(q2) + (dc6*sin(q2 + q3 + q4 - q5))/2 + d5*sin(q2 + q3 + q4);
JP(3,2) = l3*cos(q2 + q3) - (dc6*sin(q2 + q3 + q4 + q5))/2 - lc1 + l2*cos(q2) + (dc6*sin(q2 + q3 + q4 - q5))/2 + d5*sin(q2 + q3 + q4);
JP(3,3) = l3*cos(q2 + q3) - (dc6*sin(q2 + q3 + q4 + q5))/2 + l2*cos(q2) - lc2*cos(q2) + (dc6*sin(q2 + q3 + q4 - q5))/2 + d5*sin(q2 + q3 + q4);
JP(3,4) = - (dc6*sin(q2 + q3 + q4 + q5))/2 - (dc6*sin(q2 + q3 + q4 - q5))/2 - d4*sin(q2 + q3 + q4);
JP(3,5) = d4*cos(q2 + q3 + q4)*sin(q5) + d5*sin(q2 + q3 + q4)*cos(q5) - dc4*cos(q2 + q3 + q4)*sin(q5);
JP(3,6) = sin(q2 + q3 + q4)*cos(q5)*(d5 - dc5);

dp = JP*dq;

dq1 = dq(1);
dq2 = dq(2);
dq3 = dq(3);
dq4 = dq(4);
dq5 = dq(5);
%dq6 = dq(6);

dJP = zeros(3,6);

dJP(1,1) = dq1*sin(q1)*(d1 + l3*sin(q2 + q3) + l2*sin(q2) - d5*cos(q2 + q3 + q4) - dc6*sin(q2 + q3 + q4)*sin(q5)) - dq3*cos(q1)*(l3*cos(q2 + q3) + d5*sin(q2 + q3 + q4) - dc6*cos(q2 + q3 + q4)*sin(q5)) - dq4*cos(q1)*(d5*sin(q2 + q3 + q4) - dc6*cos(q2 + q3 + q4)*sin(q5)) - dq2*cos(q1)*(l3*cos(q2 + q3) + l2*cos(q2) + d5*sin(q2 + q3 + q4) - dc6*cos(q2 + q3 + q4)*sin(q5)) + dc6*dq5*sin(q2 + q3 + q4)*cos(q1)*cos(q5);
dJP(1,2) = dq1*sin(q1)*(d1 - dc1 + l3*sin(q2 + q3) + l2*sin(q2) - d5*cos(q2 + q3 + q4) - dc6*sin(q2 + q3 + q4)*sin(q5)) - dq3*cos(q1)*(l3*cos(q2 + q3) + d5*sin(q2 + q3 + q4) - dc6*cos(q2 + q3 + q4)*sin(q5)) - dq4*cos(q1)*(d5*sin(q2 + q3 + q4) - dc6*cos(q2 + q3 + q4)*sin(q5)) - dq2*cos(q1)*(l3*cos(q2 + q3) + l2*cos(q2) + d5*sin(q2 + q3 + q4) - dc6*cos(q2 + q3 + q4)*sin(q5)) + dc6*dq5*sin(q2 + q3 + q4)*cos(q1)*cos(q5);
dJP(1,3) = dc6*dq5*sin(q2 + q3 + q4)*cos(q1)*cos(q5) - dq2*cos(q1)*(l3*cos(q2 + q3) + l2*cos(q2) - lc2*cos(q2) + d5*sin(q2 + q3 + q4) - dc6*cos(q2 + q3 + q4)*sin(q5)) - dq1*sin(q1)*(lc2*sin(q2) - l2*sin(q2) - l3*sin(q2 + q3) + d5*cos(q2 + q3 + q4) + dc6*sin(q2 + q3 + q4)*sin(q5)) - dq4*cos(q1)*(d5*sin(q2 + q3 + q4) - dc6*cos(q2 + q3 + q4)*sin(q5)) - dq3*cos(q1)*(l3*cos(q2 + q3) + d5*sin(q2 + q3 + q4) - dc6*cos(q2 + q3 + q4)*sin(q5));
dJP(1,4) = dq1*l3*cos(q1)*cos(q4) - dq1*lc3*cos(q1)*cos(q4) - dc6*dq1*cos(q1)*sin(q5) - dc6*dq5*cos(q5)*sin(q1) - dq4*l3*sin(q1)*sin(q4) + dq4*lc3*sin(q1)*sin(q4) + d4*dq1*cos(q2)*cos(q3)*cos(q4)*sin(q1) + d4*dq2*cos(q1)*cos(q2)*cos(q3)*sin(q4) + d4*dq2*cos(q1)*cos(q2)*cos(q4)*sin(q3) + d4*dq2*cos(q1)*cos(q3)*cos(q4)*sin(q2) + d4*dq3*cos(q1)*cos(q2)*cos(q3)*sin(q4) + d4*dq3*cos(q1)*cos(q2)*cos(q4)*sin(q3) + d4*dq3*cos(q1)*cos(q3)*cos(q4)*sin(q2) + d4*dq4*cos(q1)*cos(q2)*cos(q3)*sin(q4) + d4*dq4*cos(q1)*cos(q2)*cos(q4)*sin(q3) + d4*dq4*cos(q1)*cos(q3)*cos(q4)*sin(q2) - d4*dq1*cos(q2)*sin(q1)*sin(q3)*sin(q4) - d4*dq1*cos(q3)*sin(q1)*sin(q2)*sin(q4) - d4*dq1*cos(q4)*sin(q1)*sin(q2)*sin(q3) - d4*dq2*cos(q1)*sin(q2)*sin(q3)*sin(q4) - d4*dq3*cos(q1)*sin(q2)*sin(q3)*sin(q4) - d4*dq4*cos(q1)*sin(q2)*sin(q3)*sin(q4) + dc6*dq1*cos(q2)*cos(q3)*cos(q4)*cos(q5)*sin(q1) + dc6*dq2*cos(q1)*cos(q2)*cos(q3)*cos(q5)*sin(q4) + dc6*dq2*cos(q1)*cos(q2)*cos(q4)*cos(q5)*sin(q3) + dc6*dq2*cos(q1)*cos(q3)*cos(q4)*cos(q5)*sin(q2) + dc6*dq3*cos(q1)*cos(q2)*cos(q3)*cos(q5)*sin(q4) + dc6*dq3*cos(q1)*cos(q2)*cos(q4)*cos(q5)*sin(q3) + dc6*dq3*cos(q1)*cos(q3)*cos(q4)*cos(q5)*sin(q2) + dc6*dq4*cos(q1)*cos(q2)*cos(q3)*cos(q5)*sin(q4) + dc6*dq4*cos(q1)*cos(q2)*cos(q4)*cos(q5)*sin(q3) + dc6*dq4*cos(q1)*cos(q3)*cos(q4)*cos(q5)*sin(q2) + dc6*dq5*cos(q1)*cos(q2)*cos(q3)*cos(q4)*sin(q5) - dc6*dq1*cos(q2)*cos(q5)*sin(q1)*sin(q3)*sin(q4) - dc6*dq1*cos(q3)*cos(q5)*sin(q1)*sin(q2)*sin(q4) - dc6*dq1*cos(q4)*cos(q5)*sin(q1)*sin(q2)*sin(q3) - dc6*dq2*cos(q1)*cos(q5)*sin(q2)*sin(q3)*sin(q4) - dc6*dq3*cos(q1)*cos(q5)*sin(q2)*sin(q3)*sin(q4) - dc6*dq4*cos(q1)*cos(q5)*sin(q2)*sin(q3)*sin(q4) - dc6*dq5*cos(q1)*cos(q2)*sin(q3)*sin(q4)*sin(q5) - dc6*dq5*cos(q1)*cos(q3)*sin(q2)*sin(q4)*sin(q5) - dc6*dq5*cos(q1)*cos(q4)*sin(q2)*sin(q3)*sin(q5);
dJP(1,5) = dq5*(d5*cos(q5)*sin(q1) - d4*sin(q2 + q3 + q4)*cos(q1)*cos(q5) - d5*cos(q2 + q3 + q4)*cos(q1)*sin(q5) + dc4*sin(q2 + q3 + q4)*cos(q1)*cos(q5)) + dq1*(d5*cos(q1)*sin(q5) - d5*cos(q2 + q3 + q4)*cos(q5)*sin(q1) + d4*sin(q2 + q3 + q4)*sin(q1)*sin(q5) - dc4*sin(q2 + q3 + q4)*sin(q1)*sin(q5)) - dq2*cos(q1)*(d4*cos(q2 + q3 + q4)*sin(q5) + d5*sin(q2 + q3 + q4)*cos(q5) - dc4*cos(q2 + q3 + q4)*sin(q5)) - dq3*cos(q1)*(d4*cos(q2 + q3 + q4)*sin(q5) + d5*sin(q2 + q3 + q4)*cos(q5) - dc4*cos(q2 + q3 + q4)*sin(q5)) - dq4*cos(q1)*(d4*cos(q2 + q3 + q4)*sin(q5) + d5*sin(q2 + q3 + q4)*cos(q5) - dc4*cos(q2 + q3 + q4)*sin(q5));
dJP(1,6) = dq1*(d5 - dc5)*(cos(q1)*sin(q5) - cos(q2 + q3 + q4)*cos(q5)*sin(q1)) + dq5*(d5 - dc5)*(cos(q5)*sin(q1) - cos(q2 + q3 + q4)*cos(q1)*sin(q5)) - dq2*sin(q2 + q3 + q4)*cos(q1)*cos(q5)*(d5 - dc5) - dq3*sin(q2 + q3 + q4)*cos(q1)*cos(q5)*(d5 - dc5) - dq4*sin(q2 + q3 + q4)*cos(q1)*cos(q5)*(d5 - dc5);

dJP(2,1) = dc6*dq5*sin(q2 + q3 + q4)*cos(q5)*sin(q1) - dq1*cos(q1)*(d1 + l3*sin(q2 + q3) + l2*sin(q2) - d5*cos(q2 + q3 + q4) - dc6*sin(q2 + q3 + q4)*sin(q5)) - dq4*sin(q1)*(d5*sin(q2 + q3 + q4) - dc6*cos(q2 + q3 + q4)*sin(q5)) - dq2*sin(q1)*(l3*cos(q2 + q3) + l2*cos(q2) + d5*sin(q2 + q3 + q4) - dc6*cos(q2 + q3 + q4)*sin(q5)) - dq3*sin(q1)*(l3*cos(q2 + q3) + d5*sin(q2 + q3 + q4) - dc6*cos(q2 + q3 + q4)*sin(q5));
dJP(2,2) = dc6*dq5*sin(q2 + q3 + q4)*cos(q5)*sin(q1) - dq4*sin(q1)*(d5*sin(q2 + q3 + q4) - dc6*cos(q2 + q3 + q4)*sin(q5)) - dq2*sin(q1)*(l3*cos(q2 + q3) + l2*cos(q2) + d5*sin(q2 + q3 + q4) - dc6*cos(q2 + q3 + q4)*sin(q5)) - dq1*cos(q1)*(d1 - dc1 + l3*sin(q2 + q3) + l2*sin(q2) - d5*cos(q2 + q3 + q4) - dc6*sin(q2 + q3 + q4)*sin(q5)) - dq3*sin(q1)*(l3*cos(q2 + q3) + d5*sin(q2 + q3 + q4) - dc6*cos(q2 + q3 + q4)*sin(q5));
dJP(2,3) = dq1*cos(q1)*(lc2*sin(q2) - l2*sin(q2) - l3*sin(q2 + q3) + d5*cos(q2 + q3 + q4) + dc6*sin(q2 + q3 + q4)*sin(q5)) - dq2*sin(q1)*(l3*cos(q2 + q3) + l2*cos(q2) - lc2*cos(q2) + d5*sin(q2 + q3 + q4) - dc6*cos(q2 + q3 + q4)*sin(q5)) - dq3*sin(q1)*(l3*cos(q2 + q3) + d5*sin(q2 + q3 + q4) - dc6*cos(q2 + q3 + q4)*sin(q5)) - dq4*sin(q1)*(d5*sin(q2 + q3 + q4) - dc6*cos(q2 + q3 + q4)*sin(q5)) + dc6*dq5*sin(q2 + q3 + q4)*cos(q5)*sin(q1);
dJP(2,4) = dc6*dq5*cos(q1)*cos(q5) + dq1*l3*cos(q4)*sin(q1) + dq4*l3*cos(q1)*sin(q4) - dq1*lc3*cos(q4)*sin(q1) - dq4*lc3*cos(q1)*sin(q4) - dc6*dq1*sin(q1)*sin(q5) - d4*dq1*cos(q1)*cos(q2)*cos(q3)*cos(q4) + d4*dq1*cos(q1)*cos(q2)*sin(q3)*sin(q4) + d4*dq1*cos(q1)*cos(q3)*sin(q2)*sin(q4) + d4*dq1*cos(q1)*cos(q4)*sin(q2)*sin(q3) + d4*dq2*cos(q2)*cos(q3)*sin(q1)*sin(q4) + d4*dq2*cos(q2)*cos(q4)*sin(q1)*sin(q3) + d4*dq2*cos(q3)*cos(q4)*sin(q1)*sin(q2) + d4*dq3*cos(q2)*cos(q3)*sin(q1)*sin(q4) + d4*dq3*cos(q2)*cos(q4)*sin(q1)*sin(q3) + d4*dq3*cos(q3)*cos(q4)*sin(q1)*sin(q2) + d4*dq4*cos(q2)*cos(q3)*sin(q1)*sin(q4) + d4*dq4*cos(q2)*cos(q4)*sin(q1)*sin(q3) + d4*dq4*cos(q3)*cos(q4)*sin(q1)*sin(q2) - d4*dq2*sin(q1)*sin(q2)*sin(q3)*sin(q4) - d4*dq3*sin(q1)*sin(q2)*sin(q3)*sin(q4) - d4*dq4*sin(q1)*sin(q2)*sin(q3)*sin(q4) - dc6*dq1*cos(q1)*cos(q2)*cos(q3)*cos(q4)*cos(q5) + dc6*dq1*cos(q1)*cos(q2)*cos(q5)*sin(q3)*sin(q4) + dc6*dq1*cos(q1)*cos(q3)*cos(q5)*sin(q2)*sin(q4) + dc6*dq1*cos(q1)*cos(q4)*cos(q5)*sin(q2)*sin(q3) + dc6*dq2*cos(q2)*cos(q3)*cos(q5)*sin(q1)*sin(q4) + dc6*dq2*cos(q2)*cos(q4)*cos(q5)*sin(q1)*sin(q3) + dc6*dq2*cos(q3)*cos(q4)*cos(q5)*sin(q1)*sin(q2) + dc6*dq3*cos(q2)*cos(q3)*cos(q5)*sin(q1)*sin(q4) + dc6*dq3*cos(q2)*cos(q4)*cos(q5)*sin(q1)*sin(q3) + dc6*dq3*cos(q3)*cos(q4)*cos(q5)*sin(q1)*sin(q2) + dc6*dq4*cos(q2)*cos(q3)*cos(q5)*sin(q1)*sin(q4) + dc6*dq4*cos(q2)*cos(q4)*cos(q5)*sin(q1)*sin(q3) + dc6*dq4*cos(q3)*cos(q4)*cos(q5)*sin(q1)*sin(q2) + dc6*dq5*cos(q2)*cos(q3)*cos(q4)*sin(q1)*sin(q5) - dc6*dq2*cos(q5)*sin(q1)*sin(q2)*sin(q3)*sin(q4) - dc6*dq3*cos(q5)*sin(q1)*sin(q2)*sin(q3)*sin(q4) - dc6*dq4*cos(q5)*sin(q1)*sin(q2)*sin(q3)*sin(q4) - dc6*dq5*cos(q2)*sin(q1)*sin(q3)*sin(q4)*sin(q5) - dc6*dq5*cos(q3)*sin(q1)*sin(q2)*sin(q4)*sin(q5) - dc6*dq5*cos(q4)*sin(q1)*sin(q2)*sin(q3)*sin(q5);
dJP(2,5) = dq1*(d5*sin(q1)*sin(q5) + d5*cos(q2 + q3 + q4)*cos(q1)*cos(q5) - d4*sin(q2 + q3 + q4)*cos(q1)*sin(q5) + dc4*sin(q2 + q3 + q4)*cos(q1)*sin(q5)) - dq5*(d5*cos(q1)*cos(q5) + d4*sin(q2 + q3 + q4)*cos(q5)*sin(q1) + d5*cos(q2 + q3 + q4)*sin(q1)*sin(q5) - dc4*sin(q2 + q3 + q4)*cos(q5)*sin(q1)) - dq2*sin(q1)*(d4*cos(q2 + q3 + q4)*sin(q5) + d5*sin(q2 + q3 + q4)*cos(q5) - dc4*cos(q2 + q3 + q4)*sin(q5)) - dq3*sin(q1)*(d4*cos(q2 + q3 + q4)*sin(q5) + d5*sin(q2 + q3 + q4)*cos(q5) - dc4*cos(q2 + q3 + q4)*sin(q5)) - dq4*sin(q1)*(d4*cos(q2 + q3 + q4)*sin(q5) + d5*sin(q2 + q3 + q4)*cos(q5) - dc4*cos(q2 + q3 + q4)*sin(q5));
dJP(2,6) = dq1*(d5 - dc5)*(sin(q1)*sin(q5) + cos(q2 + q3 + q4)*cos(q1)*cos(q5)) - dq5*(d5 - dc5)*(cos(q1)*cos(q5) + cos(q2 + q3 + q4)*sin(q1)*sin(q5)) - dq2*sin(q2 + q3 + q4)*cos(q5)*sin(q1)*(d5 - dc5) - dq3*sin(q2 + q3 + q4)*cos(q5)*sin(q1)*(d5 - dc5) - dq4*sin(q2 + q3 + q4)*cos(q5)*sin(q1)*(d5 - dc5);

dJP(3,1) = dq4*((dc6*cos(q2 + q3 + q4 - q5))/2 - (dc6*cos(q2 + q3 + q4 + q5))/2 + d5*cos(q2 + q3 + q4)) - dq3*((dc6*cos(q2 + q3 + q4 + q5))/2 + l3*sin(q2 + q3) - (dc6*cos(q2 + q3 + q4 - q5))/2 - d5*cos(q2 + q3 + q4)) - dq2*((dc6*cos(q2 + q3 + q4 + q5))/2 + l3*sin(q2 + q3) - (dc6*cos(q2 + q3 + q4 - q5))/2 + l2*sin(q2) - d5*cos(q2 + q3 + q4)) - (dc6*dq5*(cos(q2 + q3 + q4 + q5) + cos(q2 + q3 + q4 - q5)))/2;
dJP(3,2) = dq4*((dc6*cos(q2 + q3 + q4 - q5))/2 - (dc6*cos(q2 + q3 + q4 + q5))/2 + d5*cos(q2 + q3 + q4)) - dq3*((dc6*cos(q2 + q3 + q4 + q5))/2 + l3*sin(q2 + q3) - (dc6*cos(q2 + q3 + q4 - q5))/2 - d5*cos(q2 + q3 + q4)) - dq2*((dc6*cos(q2 + q3 + q4 + q5))/2 + l3*sin(q2 + q3) - (dc6*cos(q2 + q3 + q4 - q5))/2 + l2*sin(q2) - d5*cos(q2 + q3 + q4)) - (dc6*dq5*(cos(q2 + q3 + q4 + q5) + cos(q2 + q3 + q4 - q5)))/2;
dJP(3,3) = dq4*((dc6*cos(q2 + q3 + q4 - q5))/2 - (dc6*cos(q2 + q3 + q4 + q5))/2 + d5*cos(q2 + q3 + q4)) - dq3*((dc6*cos(q2 + q3 + q4 + q5))/2 + l3*sin(q2 + q3) - (dc6*cos(q2 + q3 + q4 - q5))/2 - d5*cos(q2 + q3 + q4)) - dq2*((dc6*cos(q2 + q3 + q4 + q5))/2 + l3*sin(q2 + q3) - (dc6*cos(q2 + q3 + q4 - q5))/2 + l2*sin(q2) - lc2*sin(q2) - d5*cos(q2 + q3 + q4)) - dq5*((dc6*cos(q2 + q3 + q4 + q5))/2 + (dc6*cos(q2 + q3 + q4 - q5))/2);
dJP(3,4) = - dq2*((dc6*cos(q2 + q3 + q4 + q5))/2 + (dc6*cos(q2 + q3 + q4 - q5))/2 + d4*cos(q2 + q3 + q4)) - dq3*((dc6*cos(q2 + q3 + q4 + q5))/2 + (dc6*cos(q2 + q3 + q4 - q5))/2 + d4*cos(q2 + q3 + q4)) - dq4*((dc6*cos(q2 + q3 + q4 + q5))/2 + (dc6*cos(q2 + q3 + q4 - q5))/2 + d4*cos(q2 + q3 + q4)) - (dc6*dq5*(cos(q2 + q3 + q4 + q5) - cos(q2 + q3 + q4 - q5)))/2;
dJP(3,5) = dq2*(d5*cos(q2 + q3 + q4)*cos(q5) - d4*sin(q2 + q3 + q4)*sin(q5) + dc4*sin(q2 + q3 + q4)*sin(q5)) - dq5*(dc4*cos(q2 + q3 + q4)*cos(q5) - d4*cos(q2 + q3 + q4)*cos(q5) + d5*sin(q2 + q3 + q4)*sin(q5)) + dq3*(d5*cos(q2 + q3 + q4)*cos(q5) - d4*sin(q2 + q3 + q4)*sin(q5) + dc4*sin(q2 + q3 + q4)*sin(q5)) + dq4*(d5*cos(q2 + q3 + q4)*cos(q5) - d4*sin(q2 + q3 + q4)*sin(q5) + dc4*sin(q2 + q3 + q4)*sin(q5));
dJP(3,6) = (d5 - dc5)*(dq2*cos(q2 + q3 + q4)*cos(q5) + dq3*cos(q2 + q3 + q4)*cos(q5) + dq4*cos(q2 + q3 + q4)*cos(q5) - dq5*sin(q2 + q3 + q4)*sin(q5));

ddp = dJP*ddq;

end

function m = transformacion_homogenea(DH_i)
    a_i = DH_i(1);
    alpha_i = DH_i(2);
    d_i = DH_i(3);
    theta_i = DH_i(4);
    
    ma_i = [1 0 0 a_i;
            0 1 0 0;
            0 0 1 0;
            0 0 0 1];
    
    md_i = [1 0 0 0;
            0 1 0 0;
            0 0 1 d_i;
            0 0 0 1];
    
    mtheta_i = [cos(theta_i) -sin(theta_i) 0 0;
                sin(theta_i) cos(theta_i) 0 0;
                0 0 1 0;
                0 0 0 1];
    
    malpha_i = [1 0 0 0;
                0 cos(alpha_i) -sin(alpha_i) 0;
                0 sin(alpha_i) cos(alpha_i) 0;
                0 0 0 1];
    
    m = mtheta_i * md_i * ma_i * malpha_i;

end
